simulink model "ACGen_Cycloconverter"  (R2014a)
settings: Solver=FixedStepDiscrete  StartTime=0.0  StopTime=0.6  FixedStep=Ts  RelTol=1e-3
PreLoadFcn:
  | DeadZone = 5;
  | block_angle = 90 - DeadZone;
  | Ts  = 1e-5;
  | fref = 10;
  | Eref = 4.16e3 * sqrt(2);
  | Em  = 4.16e3 * sqrt(2) / sqrt(3);
  | fao = 0;
PostLoadFcn:
  | warning off Simulink:SampleTime:IllegalIPortRateTrans
  | warning off Simulink:Commands:LoadMdlParameterizedLink
libraries: powerlib x4, powerlib_extras x2, Generator_Lib x1, simulink x1
Description:
  | Copyright 2014 The MathWorks, Inc.
settings Model: Creator=smiller  LastModifiedBy=psanghvi
settings DebuggingCC: UnderspecifiedInitializationDetection=Classic  MultiTaskRateTransMsg=warning  StateNameClashWarn=warning

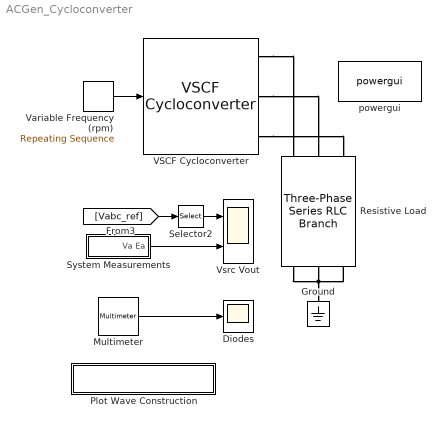
== system ACGen_Cycloconverter ==
  Diodes : Scope
      settings: TimeRange=0.005  YMin=0  YMax=20  SaveName=ScopeData5
  Ground : powerlib/Elements/Ground  LConnTagsString=a
  Multimeter : powerlib/Measurements/Multimeter  PhasorSimulation=off  OutputType=Complex  sel=[11 12]  L=16  Gain=[1 1]  yselected={'Isw1: VSCF Cycloconverter/AC Generator Cycloconverter/Phase A Cycloconverter/positive cycle','Isw2: VSCF Cycloconverter/AC Generator Cycloconverter/Phase A Cycloconverter/positive cycle'};  PSBOutputType=1  PSBequivalent=0  AxesSetting=[0,0.1,-100,100]  Display=0  SavedBlockNames=-11
  Plot Wave Construction : Subsystem
      settings: OpenFcn=Cyclo_Plot_Wave_Construction
      mask Display: disp('Plot Wave Construction');
  Resistive Load : powerlib/Elements/Three-Phase Series RLC Branch  LConnTagsString=A|B|C  RConnTagsString=A|B|C  BranchType=R  Resistance=10  Inductance=1e-3  Capacitance=1e-6  Measurements=None
  Selector2 : Selector  InputPortWidth=3
  System Measurements : Subsystem
  VSCF Cycloconverter : Generator_Lib/VSCF Cycloconverter  SystemSampleTime=-1
      link override AC Generator Cycloconverter/Phase A Cycloconverter/positive cycle: Measurements=All voltages and currents
      mask Display:
      | % This is a new mask on top of the base mask.
      | % Use "View base mask" link below to see the base mask.
      | image(imread('Gen_VSCF_Cycloconverter_IMAGE.JPG','jpg'))
      | port_label('RConn',1,'A');
      | port_label('RConn',2,'B');
      | port_label('RConn',3,'C');
      | port_label('Input',1,'Spd');
  Variable Frequency (rpm) : simulink/Sources/Repeating Sequence  rep_seq_t=[0 1 2 3 4 5 6]/5  rep_seq_y=[1 1 0.9 0.95 0.8 0.96 1]*12000
  Vsrc Vout : Scope  NumInputPorts=2
      settings: TimeRange=0.005  YMin=-200~-200  YMax=200~200  SaveName=vabc1
  powergui : powerlib/powergui  SimulationMode=Discrete  SolverType=Tustin  SampleTime=Ts  frequency=60  SPID=off  DisableSnubberDevices=off  DisableRonSwitches=off  DisableVfSwitches=off  SwTol=0  Interpol=off  DisplayEquations=off  Ts=0  methode=off  frequencyindice=0  Pbase=100e6  ErrMax=1e-4  Iterations=50  UnitsV=kV  UnitsW=MW  FunctionMessages=off  echomessages=off  HookPort=off  EnableUseOfTLC=off  x0status=blocks  RestoreLinks=warning  ResistiveCurrentMeasurement=off  Frange=[0:2:500]  Ylog=off  Xlog=on  ShowGrid=off  save=off  variable=ZData  structure=VaLoad  ZoomFFT=off  StartTime=0.3  cycles=1  DisplayStyle=2  fundamental=10  FreqAxis=on  MaxFrequency=500  frequencyindicesteady=1  RmsSteady=1  display=off
  wires:
  System Measurements/1(Va Ea) -> Vsrc Vout/2
  Selector2/1 -> Vsrc Vout/1
  [Vabc_ref] -> Selector2/1
  Variable Frequency (rpm)/1 -> VSCF Cycloconverter/1
  Multimeter/1 -> Diodes/1
  connections:
  Resistive Load/RConn1 -- Resistive Load/RConn2 -- Resistive Load/RConn3 -- Ground/LConn1
  VSCF Cycloconverter/RConn1 -- Resistive Load/LConn1
  VSCF Cycloconverter/RConn3 -- Resistive Load/LConn3
  VSCF Cycloconverter/RConn2 -- Resistive Load/LConn2

== system ACGen_Cycloconverter/Plot Wave Construction ==

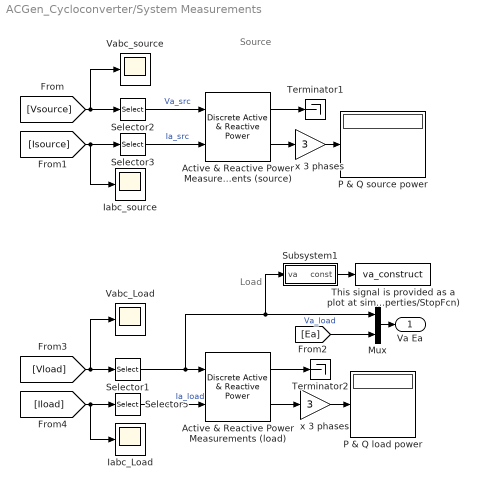
== system ACGen_Cycloconverter/System Measurements ==
  note: Source
  note: Load
  Active & Reactive Power Measurements (load) : powerlib_extras/Discrete Measurements/Discrete  Active  & Reactive  Power  Freq=400  Par_Vinit=[0 0]  Par_Iinit=[0 0]  Ts=Ts
  Active & Reactive Power Measurements (source) : powerlib_extras/Discrete Measurements/Discrete  Active  & Reactive  Power  Freq=400  Par_Vinit=[0 0]  Par_Iinit=[0 0]  Ts=Ts
  Iabc_Load : Scope
      settings: TimeRange=0.4  YMin=-1000  YMax=1000
  Iabc_source : Scope
      settings: TimeRange=0.04999710853127845  YMin=-3000  YMax=3000
  Mux : Mux  Inputs=2
  P & Q load power : Display
  P & Q source power : Display
      settings: Format=short_e
  Selector{1..3,5} (4 alike) : Selector  InputPortWidth=3
  Subsystem1 : Subsystem
  Terminator1 : Terminator
  Terminator2 : Terminator
  This signal is provided as a plot at simulation stop (See Model Properties/StopFcn) : ToWorkspace  VariableName=va_construct  SaveFormat=Structure With Time  SampleTime=-1
  Vabc_Load : Scope
      settings: TimeRange=0.4  YMin=-10000  YMax=10000  SaveName=VaLoad
  Vabc_source : Scope
      settings: TimeRange=0.050312278621926  YMin=-6000  YMax=6000  SaveName=ScopeData3
  x 3 phases : Gain  Gain=3
  "x 3 phases  " : Gain  Gain=3
  Va Ea : Outport
  wires:
  Selector2/1 -> Active & Reactive Power Measurements (source)/1  "Va_src"
  Selector3/1 -> Active & Reactive Power Measurements (source)/2  "Ia_src"
  x 3 phases/1 -> P & Q source power/1
  Mux/1 -> Va Ea/1
  [Ea] -> Mux/2
  Active & Reactive Power Measurements (source)/2 -> x 3 phases/1
  Active & Reactive Power Measurements (source)/1 -> Terminator1/1
  Subsystem1/1(const) -> This signal is provided as a plot at simulation stop (See Model Properties/StopFcn)/1
  [Vsource] -> Selector2/1, Vabc_source/1
  [Isource] -> Selector3/1, Iabc_source/1
  Selector1/1 -> Active & Reactive Power Measurements (load)/1, Subsystem1/1(va), Mux/1  "Va_load"
  Selector5/1 -> Active & Reactive Power Measurements (load)/2  "Ia_load"
  Active & Reactive Power Measurements (load)/2 -> "x 3 phases  "/1
  Active & Reactive Power Measurements (load)/1 -> Terminator2/1
  [Vload] -> Selector1/1, Vabc_Load/1
  [Iload] -> Iabc_Load/1, Selector5/1
  "x 3 phases  "/1 -> P & Q load power/1

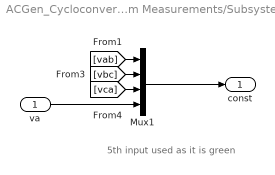
== system ACGen_Cycloconverter/System Measurements/Subsystem1 ==
  note: 5th input used as it is green
  va : Inport
  Mux1 : Mux
  const : Outport
  wires:
  [vab] -> Mux1/1
  [vbc] -> Mux1/2
  [vca] -> Mux1/3
  va/1 -> Mux1/4
  Mux1/1 -> const/1
